simulink model "LAB05"  (R2014a)
settings: Solver=ode1  StartTime=0.0  StopTime=20  FixedStep=0.002  RelTol=1e-3
undefined symbols (not defined in the file): HIL, qc_get_step_size
libraries: quarc_library x4
settings Model: SimulationMode=external  ExtModeTrigDuration=5000  Creator=gstroe  LastModifiedBy=gstroe
settings SolverCC: PositivePriorityOrder=on
settings DataIOCC: InspectSignalLogs=on
settings RTWCC: SystemTargetFile=quarc_win64.tlc  TemplateMakefile=quarc_default_tmf  Description=QUARC Win64 Target  ProcessScript=quarc_win64_make_rtw_hook
settings STFCustomTargetCC: CombineOutputUpdateFcns=on  GRTInterface=off
settings GRTTargetCC: ParMdlRefBuildCompliant=off  CompOptLevelCompliant=off  MatFileLogging=off  CPPClassGenCompliant=off  ExtMode=on  ExtModeMexFile=quarc_comm

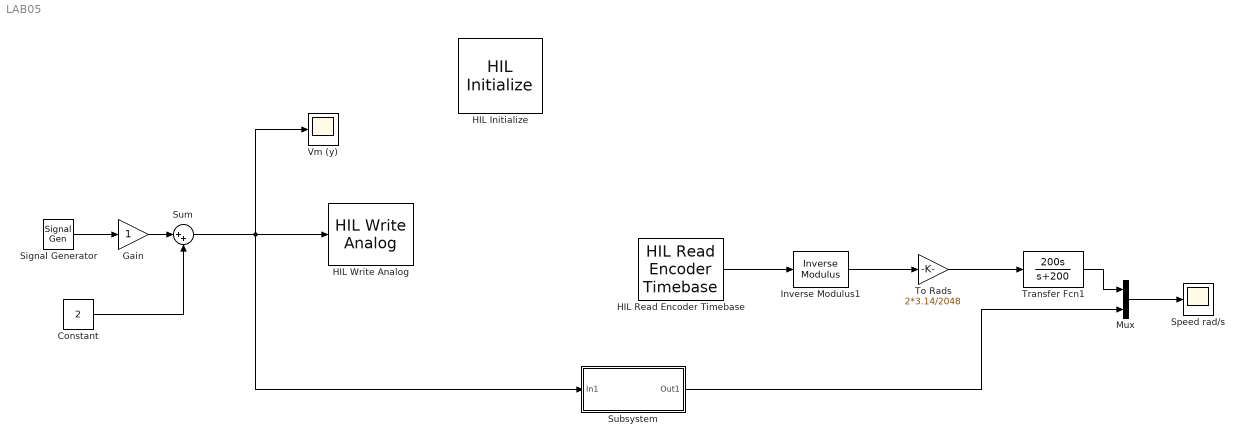
== system LAB05 ==
  Constant : Constant  Value=2
  Gain : Gain
  HIL Initialize : quarc_library/Data Acquisition/Generic/Configuration/HIL Initialize  Priority=-99  object_name=HIL-1  board_type=qube_servo_usb  board_number=0  board_options=d0=pwm;d1=pwm;led=auto;update_rate=normal;decimation=1  exclusive=off  active=off  hardware_clocks=[0]  clock_modes=[]  initial_clock_frequencies=[]  set_clock_params_at_start=off  set_clock_params_at_switch_in=off  set_clock_frequencies_at_start=off  set_clock_frequencies_at_switch_in=off  analog_input_channels=[]  analog_input_maximums=[]  analog_input_minimums=[]  set_analog_input_params_at_start=off  set_analog_input_params_at_switch_in=off  analog_output_channels=[0:1]  analog_output_maximums=10  analog_output_minimums=-10  initial_analog_outputs=[0]  final_analog_outputs=[0]  watchdog_analog_outputs=0  set_analog_output_params_at_start=on  set_analog_output_params_at_switch_in=off  set_analog_outputs_at_start=on  set_analog_outputs_at_switch_in=off  set_analog_outputs_at_terminate=on  set_analog_outputs_at_switch_out=off  set_analog_outputs_on_watchdog=off  digital_input_channels=[]  digital_output_channels=[]  digital_output_configuration=[]  initial_digital_outputs=[]  final_digital_outputs=[]  watchdog_digital_outputs=[]  set_digital_output_params_at_start=off  set_digital_output_params_at_switch_in=off  set_digital_outputs_at_start=off  set_digital_outputs_at_switch_in=off  set_digital_outputs_at_terminate=off  set_digital_outputs_at_switch_out=off  set_digital_outputs_on_watchdog=off  encoder_channels=[0:1]  quadrature=[4]  encoder_filter_frequency=[]  initial_encoder_counts=[0]  set_encoder_params_at_start=on  set_encoder_params_at_switch_in=off  set_encoder_counts_at_start=on  set_encoder_counts_at_switch_in=off  pwm_channels=[]  pwm_modes=[]  pwm_frequency=[]  pwm_configuration=[]  pwm_alignment=[]  pwm_polarity=[]  pwm_leading_deadband=[]  pwm_trailing_deadband=[]  initial_pwm_outputs=[]  final_pwm_outputs=[]  watchdog_pwm_outputs=[]  set_pwm_params_at_start=off  set_pwm_params_at_switch_in=off  set_pwm_outputs_at_start=off  set_pwm_outputs_at_switch_in=off  set_pwm_outputs_at_terminate=off  set_pwm_outputs_at_switch_out=off  set_pwm_outputs_on_watchdog=off  other_output_channels=[]  initial_other_outputs=[]  final_other_outputs=[]  watchdog_other_outputs=[]  set_other_outputs_at_start=off  set_other_outputs_at_switch_in=off  set_other_outputs_at_terminate=off  set_other_outputs_at_switch_out=off  set_other_outputs_on_watchdog=off
  HIL Read Encoder Timebase : quarc_library/Data Acquisition/Generic/Timebases/HIL Read Encoder Timebase  object_name=HIL-1  clock=0  channels=0  samples_in_buffer=max(ceil(1/qc_get_step_size), 1)  active=on  vector_output=off  data_type_mode=Inherit via back propagation  data_type=double
  HIL Write Analog : quarc_library/Data Acquisition/Generic/Immediate I//O/HIL Write Analog  object_name=HIL-1  channels=0  sample_time=-1  active=off  vector_input=off
  Inverse Modulus1 : quarc_library/Discontinuities/Inverse Modulus  modulus=2^16  output_derivative=off  output_revolutions=off  max_x=Inf  min_x=-Inf
  Mux : Mux  Inputs=2
  Signal Generator : SignalGenerator  WaveForm=square  Units=rad/sec
  Speed rad/s : Scope
      settings: YMin=0  YMax=75  SaveName=data_Wm
  Subsystem : Subsystem
  Sum : Sum  Inputs=|++
  To Rads : Gain  Gain=2*3.14/2048
  Transfer Fcn1 : TransferFcn  Numerator=[200 0]  Denominator=[1 200]
  Vm (y) : Scope
      settings: SaveName=data_Vm
  wires:
  HIL Read Encoder Timebase/1 -> Inverse Modulus1/1
  Inverse Modulus1/1 -> To Rads/1
  Sum/1 -> HIL Write Analog/1, Subsystem/1(In1), Vm (y)/1
  To Rads/1 -> Transfer Fcn1/1
  Transfer Fcn1/1 -> Mux/1
  Mux/1 -> Speed rad/s/1
  Subsystem/1(Out1) -> Mux/2
  Gain/1 -> Sum/1
  Signal Generator/1 -> Gain/1
  Constant/1 -> Sum/2

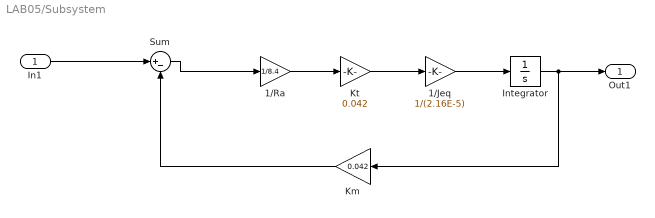
== system LAB05/Subsystem ==
  In1 : Inport
  1/Jeq : Gain  Gain=1/(2.16E-5)
  1/Ra : Gain  Gain=1/8.4
  Integrator : Integrator
  "Km " : Gain  Gain=0.042
  Kt : Gain  Gain=0.042
  Sum : Sum  Inputs=|+-
  Out1 : Outport
  wires:
  In1/1 -> Sum/1
  Sum/1 -> 1/Ra/1
  1/Ra/1 -> Kt/1
  Kt/1 -> 1/Jeq/1
  Integrator/1 -> "Km "/1, Out1/1
  "Km "/1 -> Sum/2
  1/Jeq/1 -> Integrator/1
